simulink model "Complete"  (R2016a)
settings: Solver=VariableStepAuto  StartTime=0.0  StopTime=10.0  RelTol=1e-3
values from neighbouring files (symbols this model uses):
  m = sqrt(px^2+py^2)-l5*cosd(theta234)    [GUI_robot.m]
undefined symbols (not defined in the file or in its folder): Assem1, Khop3, Khop_1, Khop_2, Khop_4, Khop_5, Khop_6, RootGround, RootPart
libraries: mblibv1 x21, simulink x5
settings Model: Creator=Loc  LastModifiedBy=Loc
settings GRTTargetCC: GeneratePreprocessorConditionals=Use local settings
settings SimMechanicsCC: VisOnUpdateDiagram=on  VisDuringSimulation=on

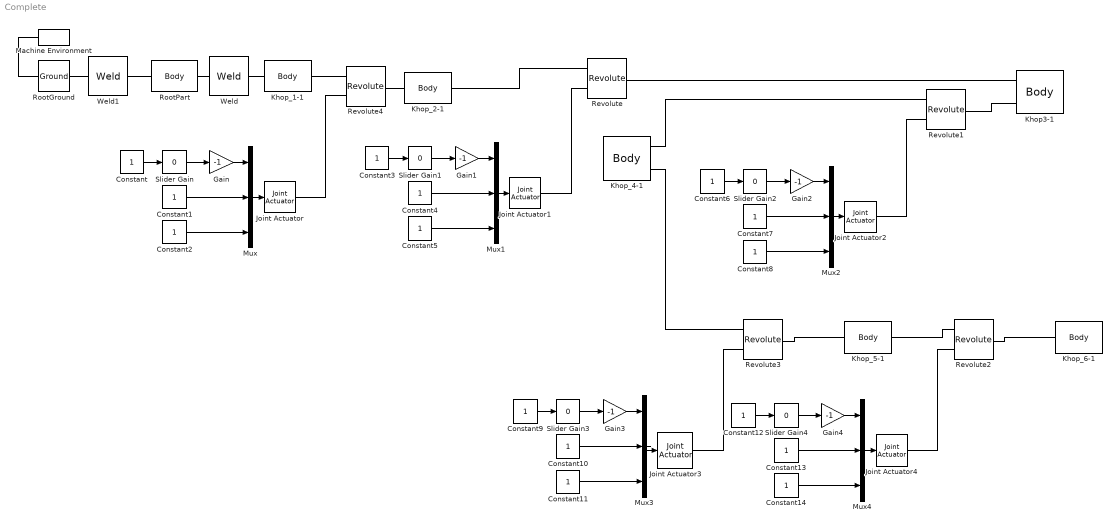
== system Complete ==
  Constant{,1..14} (15 alike) : Constant
  Gain{,1..4} (5 alike) : Gain  Gain=-1
  Joint Actuator{,1..4} (5 alike) : mblibv1/Sensors &  Actuators/Joint Actuator  UpdateFromCAD=off  PhysicalDomain=Mechanical  PortType=blob  ActuationStyle=Motion  AngleUnits=deg  ArcVelocityUnits=deg/s  ArcAccelerationUnits=deg/s^2  CoordPositionUnits=m  VelocityUnits=m/s  AccelerationUnits=m/s^2  ForceUnits=N  TorqueUnits=N*m  ActiveIO=off  Width=3  DialogClass=MechanicalActuatorBlock  Primitive=R1  ReferenceFrame=Absolute (World)
  Khop3-1 : mblibv1/Bodies/Body  LConnTagsString=CS2|CS3  UpdateFromCAD=on  PMImportedID=Khop3-1  DialogClass=MechanicalBodyBlock  Mass=28.5602  MassUnits=kg  InertiaUnits=kg*m^2  Inertia=[0.0878795,-2.92465e-12,0.0804836;-2.92465e-12,0.798937,0;0.0804836,0,0.759016]  Shape=Cylinder  ShapeDims=[1 1]  ShapeUnits=m  ShapeUse=false  Density=1  DensityUnits=kg/m^3  DensityUse=false  GraphicsMode=GFXFILE  GraphicsFileName=Assem1 - Khop3-1.STL  BodyColorSelMode=COLORPALETTE  BodyColor=[0.647059;0.619608;0.588235]  AttachedToCS=CS1  CG=Right$CG$[0.297025 -0.104442 0.799]$WORLD$WORLD$m$[1 4.11525e-12 0;0 0 -1;-4.11525e-12 1 0]$3x3 Transform$rad$WORLD$false$Khop3-1::CG(AUTOGEN)  WorkingFrames=Right$CS1$[0 0 0.799]$WORLD$WORLD$m$[1 4.11525e-12 0;0 0 -1;-4.11525e-12 1 0]$3x3 Transform$rad$WORLD$false$Khop3-1::CS1(AUTOGEN)#Left$CS2$[0 -0.06263 0.799]$WORLD$WORLD$m$[1 0 0;0 1 0;0 0 1]$3x3 Transform$rad$WORLD$true$Khop3-1:-:Khop_2-1::Khop3-1(AUTOGEN)#Left$CS3$[0.44 0.02737 0.799]$WORLD$WORLD$m$[1 0 0;0 1 0;0 0 1]$3x3 Transform$rad$WORLD$true$Khop3-1:-:Khop_4-1::Khop3-1(AUTOGEN)  CGPos=[0.297025 -0.104442 0.799]  CGRot=[1 4.11525e-12 0;0 0 -1;-4.11525e-12 1 0]  CS0Pos=[]  CS0Rot=[]  CS1Pos=[0 0 0.799]  CS1Rot=[1 4.11525e-12 0;0 0 -1;-4.11525e-12 1 0]  CS2Pos=[0 -0.06263 0.799]  CS2Rot=[1 0 0;0 1 0;0 0 1]  CS3Pos=[0.44 0.02737 0.799]  CS3Rot=[1 0 0;0 1 0;0 0 1]  CS4Pos=[]  CS4Rot=[]  CS5Pos=[]  CS5Rot=[]  CS6Pos=[]  CS6Rot=[]  CS7Pos=[]  CS7Rot=[]  CS8Pos=[]  CS8Rot=[]  CS9Pos=[]  CS9Rot=[]  CS10Pos=[]  CS10Rot=[]  CS11Pos=[]  CS11Rot=[]  CS12Pos=[]  CS12Rot=[]  CS13Pos=[]  CS13Rot=[]  CS14Pos=[]  CS14Rot=[]  CS15Pos=[]  CS15Rot=[]  CS16Pos=[]  CS16Rot=[]  CS17Pos=[]  CS17Rot=[]  CS18Pos=[]  CS18Rot=[]  CS19Pos=[]  CS19Rot=[]  CS20Pos=[]  CS20Rot=[]
  Khop_1-1 : mblibv1/Bodies/Body  LConnTagsString=CS2  RConnTagsString=CS3  UpdateFromCAD=on  PMImportedID=Khop_1-1  DialogClass=MechanicalBodyBlock  Mass=93.2643  MassUnits=kg  InertiaUnits=kg*m^2  Inertia=[3.0925,1.5658e-06,-3.82573e-06;1.5658e-06,3.15469,0.00058353;-3.82573e-06,0.00058353,1.19472]  Shape=Cylinder  ShapeDims=[1 1]  ShapeUnits=m  ShapeUse=false  Density=1  DensityUnits=kg/m^3  DensityUse=false  GraphicsMode=GFXFILE  GraphicsFileName=Assem1 - Khop_1-1.STL  BodyColorSelMode=COLORPALETTE  BodyColor=[0.647059;0.619608;0.588235]  AttachedToCS=CS1  CG=Right$CG$[2.16533e-07 0.00269678 0.260737]$WORLD$WORLD$m$[1 0 0;0 1 0;0 0 1]$3x3 Transform$rad$WORLD$false$Khop_1-1::CG(AUTOGEN)  WorkingFrames=Right$CS1$[0 0 0]$WORLD$WORLD$m$[1 0 0;0 1 0;0 0 1]$3x3 Transform$rad$WORLD$false$Khop_1-1::CS1(AUTOGEN)#Left$CS2$[2.16533e-07 0.00269678 0.260737]$WORLD$WORLD$m$[1 0 0;0 1 0;0 0 1]$3x3 Transform$rad$WORLD$true$Assem1/RootPart:-:Khop_1-1::Khop_1-1(AUTOGEN)#Right$CS3$[0 0 0.56]$WORLD$WORLD$m$[1 0 0;0 1 0;0 0 1]$3x3 Transform$rad$WORLD$true$Khop_1-1:-:Khop_2-1::Khop_1-1(AUTOGEN)  CGPos=[2.16533e-07 0.00269678 0.260737]  CGRot=[1 0 0;0 1 0;0 0 1]  CS0Pos=[]  CS0Rot=[]  CS1Pos=[0 0 0]  CS1Rot=[1 0 0;0 1 0;0 0 1]  CS2Pos=[2.16533e-07 0.00269678 0.260737]  CS2Rot=[1 0 0;0 1 0;0 0 1]  CS3Pos=[0 0 0.56]  CS3Rot=[1 0 0;0 1 0;0 0 1]  CS4Pos=[]  CS4Rot=[]  CS5Pos=[]  CS5Rot=[]  CS6Pos=[]  CS6Rot=[]  CS7Pos=[]  CS7Rot=[]  CS8Pos=[]  CS8Rot=[]  CS9Pos=[]  CS9Rot=[]  CS10Pos=[]  CS10Rot=[]  CS11Pos=[]  CS11Rot=[]  CS12Pos=[]  CS12Rot=[]  CS13Pos=[]  CS13Rot=[]  CS14Pos=[]  CS14Rot=[]  CS15Pos=[]  CS15Rot=[]  CS16Pos=[]  CS16Rot=[]  CS17Pos=[]  CS17Rot=[]  CS18Pos=[]  CS18Rot=[]  CS19Pos=[]  CS19Rot=[]  CS20Pos=[]  CS20Rot=[]
  Khop_2-1 : mblibv1/Bodies/Body  LConnTagsString=CS3  RConnTagsString=CS2  UpdateFromCAD=on  PMImportedID=Khop_2-1  DialogClass=MechanicalBodyBlock  Mass=43.0074  MassUnits=kg  InertiaUnits=kg*m^2  Inertia=[0.706478,-0.00179507,0.000463712;-0.00179507,0.681014,-0.0327393;0.000463712,-0.0327393,0.359804]  Shape=Cylinder  ShapeDims=[1 1]  ShapeUnits=m  ShapeUse=false  Density=1  DensityUnits=kg/m^3  DensityUse=false  GraphicsMode=GFXFILE  GraphicsFileName=Assem1 - Khop_2-1.STL  BodyColorSelMode=COLORPALETTE  BodyColor=[0.647059;0.619608;0.588235]  AttachedToCS=CS1  CG=Right$CG$[0.00220338 0.00616855 0.703759]$WORLD$WORLD$m$[1 0 0;0 1 0;0 0 1]$3x3 Transform$rad$WORLD$false$Khop_2-1::CG(AUTOGEN)  WorkingFrames=Right$CS1$[0 0 0.56]$WORLD$WORLD$m$[1 0 0;0 1 0;0 0 1]$3x3 Transform$rad$WORLD$false$Khop_2-1::CS1(AUTOGEN)#Right$CS2$[0 -0.06263 0.799]$WORLD$WORLD$m$[1 0 0;0 1 0;0 0 1]$3x3 Transform$rad$WORLD$true$Khop3-1:-:Khop_2-1::Khop_2-1(AUTOGEN)#Left$CS3$[0 0 0.56]$WORLD$WORLD$m$[1 0 0;0 1 0;0 0 1]$3x3 Transform$rad$WORLD$true$Khop_1-1:-:Khop_2-1::Khop_2-1(AUTOGEN)  CGPos=[0.00220338 0.00616855 0.703759]  CGRot=[1 0 0;0 1 0;0 0 1]  CS0Pos=[]  CS0Rot=[]  CS1Pos=[0 0 0.56]  CS1Rot=[1 0 0;0 1 0;0 0 1]  CS2Pos=[0 -0.06263 0.799]  CS2Rot=[1 0 0;0 1 0;0 0 1]  CS3Pos=[0 0 0.56]  CS3Rot=[1 0 0;0 1 0;0 0 1]  CS4Pos=[]  CS4Rot=[]  CS5Pos=[]  CS5Rot=[]  CS6Pos=[]  CS6Rot=[]  CS7Pos=[]  CS7Rot=[]  CS8Pos=[]  CS8Rot=[]  CS9Pos=[]  CS9Rot=[]  CS10Pos=[]  CS10Rot=[]  CS11Pos=[]  CS11Rot=[]  CS12Pos=[]  CS12Rot=[]  CS13Pos=[]  CS13Rot=[]  CS14Pos=[]  CS14Rot=[]  CS15Pos=[]  CS15Rot=[]  CS16Pos=[]  CS16Rot=[]  CS17Pos=[]  CS17Rot=[]  CS18Pos=[]  CS18Rot=[]  CS19Pos=[]  CS19Rot=[]  CS20Pos=[]  CS20Rot=[]
  Khop_4-1 : mblibv1/Bodies/Body  RConnTagsString=CS2|CS3  UpdateFromCAD=on  PMImportedID=Khop_4-1  DialogClass=MechanicalBodyBlock  Mass=73.6569  MassUnits=kg  InertiaUnits=kg*m^2  Inertia=[0.423966,0,-0.51029;0,4.50795,0;-0.51029,0,4.22608]  Shape=Cylinder  ShapeDims=[1 1]  ShapeUnits=m  ShapeUse=false  Density=1  DensityUnits=kg/m^3  DensityUse=false  GraphicsMode=GFXFILE  GraphicsFileName=Assem1 - Khop_4-1.STL  BodyColorSelMode=COLORPALETTE  BodyColor=[0.647059;0.619608;0.588235]  AttachedToCS=CS1  CG=Right$CG$[0.439598 0.124568 0.799]$WORLD$WORLD$m$[1 0 0;0 0 -1;0 1 0]$3x3 Transform$rad$WORLD$false$Khop_4-1::CG(AUTOGEN)  WorkingFrames=Right$CS1$[0.44 0 0.799]$WORLD$WORLD$m$[1 0 0;0 0 -1;0 1 0]$3x3 Transform$rad$WORLD$false$Khop_4-1::CS1(AUTOGEN)#Right$CS2$[0.44 0.02737 0.799]$WORLD$WORLD$m$[1 0 0;0 1 0;0 0 1]$3x3 Transform$rad$WORLD$true$Khop3-1:-:Khop_4-1::Khop_4-1(AUTOGEN)#Right$CS3$[0.9441 0.03237 0.799]$WORLD$WORLD$m$[1 0 0;0 1 0;0 0 1]$3x3 Transform$rad$WORLD$true$Khop_4-1:-:Khop_5-1::Khop_4-1(AUTOGEN)  CGPos=[0.439598 0.124568 0.799]  CGRot=[1 0 0;0 0 -1;0 1 0]  CS0Pos=[]  CS0Rot=[]  CS1Pos=[0.44 0 0.799]  CS1Rot=[1 0 0;0 0 -1;0 1 0]  CS2Pos=[0.44 0.02737 0.799]  CS2Rot=[1 0 0;0 1 0;0 0 1]  CS3Pos=[0.9441 0.03237 0.799]  CS3Rot=[1 0 0;0 1 0;0 0 1]  CS4Pos=[]  CS4Rot=[]  CS5Pos=[]  CS5Rot=[]  CS6Pos=[]  CS6Rot=[]  CS7Pos=[]  CS7Rot=[]  CS8Pos=[]  CS8Rot=[]  CS9Pos=[]  CS9Rot=[]  CS10Pos=[]  CS10Rot=[]  CS11Pos=[]  CS11Rot=[]  CS12Pos=[]  CS12Rot=[]  CS13Pos=[]  CS13Rot=[]  CS14Pos=[]  CS14Rot=[]  CS15Pos=[]  CS15Rot=[]  CS16Pos=[]  CS16Rot=[]  CS17Pos=[]  CS17Rot=[]  CS18Pos=[]  CS18Rot=[]  CS19Pos=[]  CS19Rot=[]  CS20Pos=[]  CS20Rot=[]
  Khop_5-1 : mblibv1/Bodies/Body  LConnTagsString=CS3  RConnTagsString=CS2  UpdateFromCAD=on  PMImportedID=Khop_5-1  DialogClass=MechanicalBodyBlock  Mass=4.709  MassUnits=kg  InertiaUnits=kg*m^2  Inertia=[0.00474663,-1.83096e-10,7.23019e-05;-1.83096e-10,0.00586928,-6.91179e-10;7.23019e-05,-6.91179e-10,0.00667741]  Shape=Cylinder  ShapeDims=[1 1]  ShapeUnits=m  ShapeUse=false  Density=1  DensityUnits=kg/m^3  DensityUse=false  GraphicsMode=GFXFILE  GraphicsFileName=Assem1 - Khop_5-1.STL  BodyColorSelMode=COLORPALETTE  BodyColor=[0.647059;0.619608;0.588235]  AttachedToCS=CS1  CG=Right$CG$[0.948329 -0.00363644 0.799]$WORLD$WORLD$m$[1 0 0;0 0 -1;0 1 0]$3x3 Transform$rad$WORLD$false$Khop_5-1::CG(AUTOGEN)  WorkingFrames=Right$CS1$[0.9441 0 0.799]$WORLD$WORLD$m$[1 0 0;0 0 -1;0 1 0]$3x3 Transform$rad$WORLD$false$Khop_5-1::CS1(AUTOGEN)#Right$CS2$[0.9941 -5e-06 0.799]$WORLD$WORLD$m$[1 0 0;0 1 0;0 0 1]$3x3 Transform$rad$WORLD$true$Khop_5-1:-:Khop_6-1::Khop_5-1(AUTOGEN)#Left$CS3$[0.9441 0.03237 0.799]$WORLD$WORLD$m$[1 0 0;0 1 0;0 0 1]$3x3 Transform$rad$WORLD$true$Khop_4-1:-:Khop_5-1::Khop_5-1(AUTOGEN)  CGPos=[0.948329 -0.00363644 0.799]  CGRot=[1 0 0;0 0 -1;0 1 0]  CS0Pos=[]  CS0Rot=[]  CS1Pos=[0.9441 0 0.799]  CS1Rot=[1 0 0;0 0 -1;0 1 0]  CS2Pos=[0.9941 -5e-06 0.799]  CS2Rot=[1 0 0;0 1 0;0 0 1]  CS3Pos=[0.9441 0.03237 0.799]  CS3Rot=[1 0 0;0 1 0;0 0 1]  CS4Pos=[]  CS4Rot=[]  CS5Pos=[]  CS5Rot=[]  CS6Pos=[]  CS6Rot=[]  CS7Pos=[]  CS7Rot=[]  CS8Pos=[]  CS8Rot=[]  CS9Pos=[]  CS9Rot=[]  CS10Pos=[]  CS10Rot=[]  CS11Pos=[]  CS11Rot=[]  CS12Pos=[]  CS12Rot=[]  CS13Pos=[]  CS13Rot=[]  CS14Pos=[]  CS14Rot=[]  CS15Pos=[]  CS15Rot=[]  CS16Pos=[]  CS16Rot=[]  CS17Pos=[]  CS17Rot=[]  CS18Pos=[]  CS18Rot=[]  CS19Pos=[]  CS19Rot=[]  CS20Pos=[]  CS20Rot=[]
  Khop_6-1 : mblibv1/Bodies/Body  LConnTagsString=CS2  UpdateFromCAD=on  PMImportedID=Khop_6-1  DialogClass=MechanicalBodyBlock  Mass=0.55017  MassUnits=kg  InertiaUnits=kg*m^2  Inertia=[0.00027463,1.36707e-09,1.43175e-08;1.36707e-09,0.000172309,1.62781e-09;1.43175e-08,1.62781e-09,0.000389442]  Shape=Cylinder  ShapeDims=[1 1]  ShapeUnits=m  ShapeUse=false  Density=1  DensityUnits=kg/m^3  DensityUse=false  GraphicsMode=GFXFILE  GraphicsFileName=Assem1 - Khop_6-1.STL  BodyColorSelMode=COLORPALETTE  BodyColor=[0.647059;0.619608;0.588235]  AttachedToCS=CS1  CG=Right$CG$[1.0342 -4.6001e-06 0.798996]$WORLD$WORLD$m$[0 0 1;0 -1 0;1 0 0]$3x3 Transform$rad$WORLD$false$Khop_6-1::CG(AUTOGEN)  WorkingFrames=Right$CS1$[0.9441 -5e-06 0.799]$WORLD$WORLD$m$[0 0 1;0 -1 0;1 0 0]$3x3 Transform$rad$WORLD$false$Khop_6-1::CS1(AUTOGEN)#Left$CS2$[0.9941 -5e-06 0.799]$WORLD$WORLD$m$[1 0 0;0 1 0;0 0 1]$3x3 Transform$rad$WORLD$true$Khop_5-1:-:Khop_6-1::Khop_6-1(AUTOGEN)  CGPos=[1.0342 -4.6001e-06 0.798996]  CGRot=[0 0 1;0 -1 0;1 0 0]  CS0Pos=[]  CS0Rot=[]  CS1Pos=[0.9441 -5e-06 0.799]  CS1Rot=[0 0 1;0 -1 0;1 0 0]  CS2Pos=[0.9941 -5e-06 0.799]  CS2Rot=[1 0 0;0 1 0;0 0 1]  CS3Pos=[]  CS3Rot=[]  CS4Pos=[]  CS4Rot=[]  CS5Pos=[]  CS5Rot=[]  CS6Pos=[]  CS6Rot=[]  CS7Pos=[]  CS7Rot=[]  CS8Pos=[]  CS8Rot=[]  CS9Pos=[]  CS9Rot=[]  CS10Pos=[]  CS10Rot=[]  CS11Pos=[]  CS11Rot=[]  CS12Pos=[]  CS12Rot=[]  CS13Pos=[]  CS13Rot=[]  CS14Pos=[]  CS14Rot=[]  CS15Pos=[]  CS15Rot=[]  CS16Pos=[]  CS16Rot=[]  CS17Pos=[]  CS17Rot=[]  CS18Pos=[]  CS18Rot=[]  CS19Pos=[]  CS19Rot=[]  CS20Pos=[]  CS20Rot=[]
  Machine Environment : mblibv1/Bodies/Machine Environment  PortType=env  PhysicalDomain=Mechanical  DialogTemplateClass=MECH.MachineEnvironment  SyncWhenCopied=off  Gravity=[0 -9.81 0]  GravityUnits=m/s^2  GravityAsSignal=off  Dimensionality=Auto-detect  AnalysisType=Forward dynamics  LinearAssemblyTolerance=1e-3  LinearAssemblyToleranceUnits=m  AngularAssemblyTolerance=1e-3  AngularAssemblyToleranceUnits=rad  ConstraintSolverType=Stabilizing  ConstraintRelTolerance=1e-4  ConstraintAbsTolerance=1e-4  UseRobustSingularityHandling=off  RedundancyAnalysisToleranceType=Automatically select tolerance  RedundancyAnalysisTolerance=1e-14  StatePerturbationType=Fixed  PerturbationSize=1e-5  VisualizeMachine=on  BodyVisualizationType=Use model default body geometries  BodyColorSelMode=Use model default  DefaultBodyColor=[1 0 0]
  Mux{,1..4} (5 alike) : Mux  Inputs=3
  Revolute : mblibv1/Joints/Revolute  LConnTagsString=__newl0|SA1  RConnTagsString=__newr0  UpdateFromCAD=on  PMImportedID=Khop3-1:-:Khop_2-1  NumSAPorts=1  CutJoint=off  MarkAsCut=off  Primitives=prismatic  PrimitiveProps=R1$World$[0,1,0]$revolute  DialogClass=JointBlock  R1Axis=[0,1,0]
  Revolute1 : mblibv1/Joints/Revolute  LConnTagsString=__newl0|SA1  RConnTagsString=__newr0  UpdateFromCAD=on  PMImportedID=Khop3-1:-:Khop_4-1  NumSAPorts=1  CutJoint=off  MarkAsCut=off  Primitives=prismatic  PrimitiveProps=R1$World$[0,-1,0]$revolute  DialogClass=JointBlock  R1Axis=[0,-1,0]
  Revolute2 : mblibv1/Joints/Revolute  LConnTagsString=__newl0|SA1  RConnTagsString=__newr0  UpdateFromCAD=on  PMImportedID=Khop_5-1:-:Khop_6-1  NumSAPorts=1  CutJoint=off  MarkAsCut=off  Primitives=prismatic  PrimitiveProps=R1$World$[1,0,0]$revolute  DialogClass=JointBlock  R1Axis=[1,0,0]
  Revolute3 : mblibv1/Joints/Revolute  LConnTagsString=__newl0|SA1  RConnTagsString=__newr0  UpdateFromCAD=on  PMImportedID=Khop_4-1:-:Khop_5-1  NumSAPorts=1  CutJoint=off  MarkAsCut=off  Primitives=prismatic  PrimitiveProps=R1$World$[0,1,0]$revolute  DialogClass=JointBlock  R1Axis=[0,1,0]
  Revolute4 : mblibv1/Joints/Revolute  LConnTagsString=__newl0|SA1  RConnTagsString=__newr0  UpdateFromCAD=on  PMImportedID=Khop_1-1:-:Khop_2-1  NumSAPorts=1  CutJoint=off  MarkAsCut=off  Primitives=prismatic  PrimitiveProps=R1$World$[0,0,1]$revolute  DialogClass=JointBlock  R1Axis=[0,0,1]
  RootGround : mblibv1/Bodies/Ground  UpdateFromCAD=on  PMImportedID=RootGround  LeftPortType=env  RightPortType=workingframe  PhysicalDomain=Mechanical  DialogClass=GroundBlock  CoordPosition=[0.188687,0.0274551,0.576242]  CoordPositionUnits=m  StateVectorMgrId=0  MachineId=[1 0]  ShowEnvPort=on  ParameterChecksum=[412524562, 1506260019, 1145559585, 447755277]  TopologyChecksum=[1665056996, 376394296, 4191182034, 2231205444]
  RootPart : mblibv1/Bodies/Body  LConnTagsString=CS3  RConnTagsString=CS2  UpdateFromCAD=on  PMImportedID=Assem1/RootPart  DialogClass=MechanicalBodyBlock  Mass=0  MassUnits=kg  InertiaUnits=kg*m^2  Inertia=[0,0,0;0,0,0;0,0,0]  Shape=Cylinder  ShapeDims=[1 1]  ShapeUnits=m  ShapeUse=false  Density=1  DensityUnits=kg/m^3  DensityUse=false  GraphicsMode=MACHINE_DEFAULT  BodyColorSelMode=MACHINE_DEFAULT  BodyColor=[1;0;0]  AttachedToCS=CS1  CG=Right$CG$[0.188687 0.0274551 0.576242]$WORLD$WORLD$m$[1 0 0;0 1 0;0 0 1]$3x3 Transform$rad$WORLD$false$Assem1/RootPart::CG(AUTOGEN)  WorkingFrames=Right$CS1$[0 0 0]$WORLD$WORLD$m$[1 0 0;0 1 0;0 0 1]$3x3 Transform$rad$WORLD$false$Assem1/RootPart::CS1(AUTOGEN)#Right$CS2$[2.16533e-07 0.00269678 0.260737]$WORLD$WORLD$m$[1 0 0;0 1 0;0 0 1]$3x3 Transform$rad$WORLD$true$Assem1/RootPart:-:Khop_1-1::Assem1/RootPart(AUTOGEN)#Left$CS3$[0.188687 0.0274551 0.576242]$WORLD$WORLD$m$[1 0 0;0 1 0;0 0 1]$3x3 Transform$rad$WORLD$true$Assem1/RootPart:-:RootGround::Assem1/RootPart(AUTOGEN)  CGPos=[0.188687 0.0274551 0.576242]  CGRot=[1 0 0;0 1 0;0 0 1]  CS0Pos=[]  CS0Rot=[]  CS1Pos=[0 0 0]  CS1Rot=[1 0 0;0 1 0;0 0 1]  CS2Pos=[2.16533e-07 0.00269678 0.260737]  CS2Rot=[1 0 0;0 1 0;0 0 1]  CS3Pos=[0.188687 0.0274551 0.576242]  CS3Rot=[1 0 0;0 1 0;0 0 1]  CS4Pos=[]  CS4Rot=[]  CS5Pos=[]  CS5Rot=[]  CS6Pos=[]  CS6Rot=[]  CS7Pos=[]  CS7Rot=[]  CS8Pos=[]  CS8Rot=[]  CS9Pos=[]  CS9Rot=[]  CS10Pos=[]  CS10Rot=[]  CS11Pos=[]  CS11Rot=[]  CS12Pos=[]  CS12Rot=[]  CS13Pos=[]  CS13Rot=[]  CS14Pos=[]  CS14Rot=[]  CS15Pos=[]  CS15Rot=[]  CS16Pos=[]  CS16Rot=[]  CS17Pos=[]  CS17Rot=[]  CS18Pos=[]  CS18Rot=[]  CS19Pos=[]  CS19Rot=[]  CS20Pos=[]  CS20Rot=[]
  Slider Gain{,1..4} (5 alike) : simulink/Math Operations/Slider Gain  low=-180  gain=0  high=180
  Weld : mblibv1/Joints/Weld  LConnTagsString=__newl0  RConnTagsString=__newr0  UpdateFromCAD=on  PMImportedID=Assem1/RootPart:-:Khop_1-1  NumSAPorts=0  CutJoint=off  MarkAsCut=off  Primitives=weld  PrimitiveProps=W$WORLD$[0.57735,0.57735,0.57735]$weld  DialogClass=JointBlock  WAxis=[0.57735,0.57735,0.57735]
  Weld1 : mblibv1/Joints/Weld  LConnTagsString=__newl0  RConnTagsString=__newr0  UpdateFromCAD=on  PMImportedID=Assem1/RootPart:-:RootGround  NumSAPorts=0  CutJoint=off  MarkAsCut=off  Primitives=weld  PrimitiveProps=W$WORLD$[0.57735,0.57735,0.57735]$weld  DialogClass=JointBlock  WAxis=[0.57735,0.57735,0.57735]
  wires:
  Constant1/1 -> Mux/2
  Constant2/1 -> Mux/3
  Mux/1 -> Joint Actuator/1
  Constant/1 -> Slider Gain/1
  Gain/1 -> Mux/1
  Slider Gain/1 -> Gain/1
  Constant4/1 -> Mux1/2
  Constant5/1 -> Mux1/3
  Mux1/1 -> Joint Actuator1/1
  Constant3/1 -> Slider Gain1/1
  Gain1/1 -> Mux1/1
  Slider Gain1/1 -> Gain1/1
  Constant7/1 -> Mux2/2
  Constant8/1 -> Mux2/3
  Mux2/1 -> Joint Actuator2/1
  Constant6/1 -> Slider Gain2/1
  Gain2/1 -> Mux2/1
  Slider Gain2/1 -> Gain2/1
  Constant10/1 -> Mux3/2
  Constant11/1 -> Mux3/3
  Mux3/1 -> Joint Actuator3/1
  Constant9/1 -> Slider Gain3/1
  Gain3/1 -> Mux3/1
  Slider Gain3/1 -> Gain3/1
  Constant13/1 -> Mux4/2
  Constant14/1 -> Mux4/3
  Mux4/1 -> Joint Actuator4/1
  Constant12/1 -> Slider Gain4/1
  Gain4/1 -> Mux4/1
  Slider Gain4/1 -> Gain4/1
  connections:
  RootPart/RConn1 -- Weld/LConn1
  Weld/RConn1 -- Khop_1-1/LConn1
  Khop_2-1/RConn1 -- Revolute/LConn1
  Revolute/RConn1 -- Khop3-1/LConn1
  Khop_4-1/RConn1 -- Revolute1/LConn1
  Revolute1/RConn1 -- Khop3-1/LConn2
  Khop_5-1/RConn1 -- Revolute2/LConn1
  Revolute2/RConn1 -- Khop_6-1/LConn1
  Khop_4-1/RConn2 -- Revolute3/LConn1
  Revolute3/RConn1 -- Khop_5-1/LConn1
  Khop_1-1/RConn1 -- Revolute4/LConn1
  Revolute4/RConn1 -- Khop_2-1/LConn1
  RootGround/RConn1 -- Weld1/LConn1
  Weld1/RConn1 -- RootPart/LConn1
  RootGround/LConn1 -- Machine Environment/RConn1
  Revolute4/LConn2 -- Joint Actuator/RConn1
  Revolute/LConn2 -- Joint Actuator1/RConn1
  Revolute1/LConn2 -- Joint Actuator2/RConn1
  Revolute3/LConn2 -- Joint Actuator3/RConn1
  Revolute2/LConn2 -- Joint Actuator4/RConn1
